simulink model "ChuaMultipleSynch_MPC_2"  (R2014b)
settings: Solver=ode4  StartTime=0.0  StopTime=T  FixedStep=Ts  RelTol=1e-8
values from neighbouring files (symbols this model uses):
  mpc = MPCController(model, N)    [main_mpc.m]
  x0 = [0.02;0.05;0.04;0.0;1.0;0.0]    [PlotEig.m]    (also in main_mpc.m; main_sim.m)
undefined symbols (not defined in the file or in its folder): MPC_Controller
settings Model: Creator=gianni  LastModifiedBy=Gianni

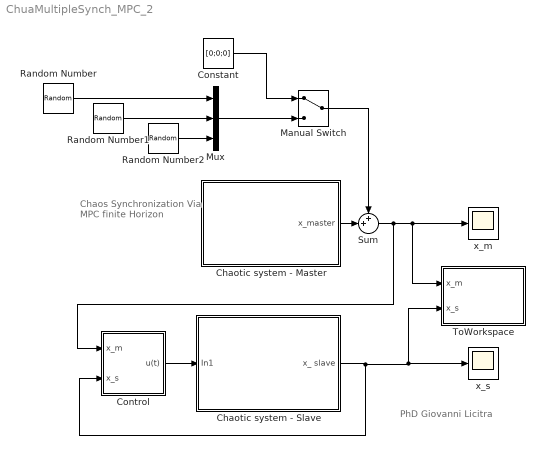
== system ChuaMultipleSynch_MPC_2 ==
  note: PhD Giovanni Licitra
  note: Chaos Synchronization
      | Via MPC finite Horizon
  Chaotic system - Master : Subsystem
      mask Display: image('Chaos.jpg')
  Chaotic system - Slave : Subsystem
      mask Display: image('Chaos.jpg')
  Constant : Constant  Value=[0;0;0]
  Control : Subsystem
  Manual Switch : ManualSwitch
  Mux : Mux  Inputs=3
  Random Number : RandomNumber  Variance=0.002
  Random Number1 : RandomNumber  Variance=0.002
  Random Number2 : RandomNumber  Variance=0.002
  Sum : Sum  Inputs=++|
  ToWorkspace : Subsystem
  x_m : Scope
      settings: YMin=-0.4  YMax=0.4
  x_s : Scope
      settings: YMin=-2
  wires:
  Control/1(u(t)) -> Chaotic system - Slave/1(In1)
  Sum/1 -> ToWorkspace/1(x_m), x_m/1, Control/1(x_m)
  Chaotic system - Slave/1(x_ slave) -> Control/2(x_s), ToWorkspace/2(x_s), x_s/1
  Mux/1 -> Manual Switch/2
  Chaotic system - Master/1(x_master) -> Sum/2
  Manual Switch/1 -> Sum/1
  Random Number/1 -> Mux/1
  Random Number1/1 -> Mux/2
  Random Number2/1 -> Mux/3
  Constant/1 -> Manual Switch/1

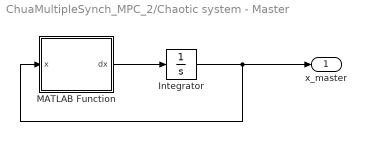
== system ChuaMultipleSynch_MPC_2/Chaotic system - Master ==
  Integrator : Integrator  InitialCondition=x0([1:3])
  MATLAB Function : MATLAB Function  TreatAsAtomicUnit=on
  x_master : Outport
  wires:
  Integrator/1 -> x_master/1, MATLAB Function/1(x)
  MATLAB Function/1(dx) -> Integrator/1

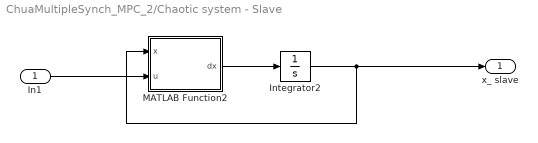
== system ChuaMultipleSynch_MPC_2/Chaotic system - Slave ==
  In1 : Inport
  Integrator2 : Integrator  InitialCondition=x0([4:6])
  MATLAB Function2 : MATLAB Function  TreatAsAtomicUnit=on
  x_ slave : Outport
  wires:
  MATLAB Function2/1(dx) -> Integrator2/1
  In1/1 -> MATLAB Function2/2(u)
  Integrator2/1 -> x_ slave/1, MATLAB Function2/1(x)

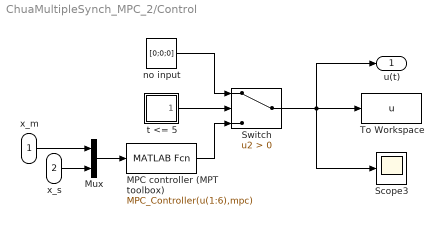
== system ChuaMultipleSynch_MPC_2/Control ==
  x_m : Inport
  x_s : Inport  Port=2
  MPC controller (MPT toolbox) : MATLABFcn  MATLABFcn=MPC_Controller(u(1:6),mpc)
  Mux : Mux  Inputs=2
  Scope3 : Scope
      settings: YMin=-20  YMax=20  SaveName=ScopeData3
  Switch : Switch  Criteria=u2 > Threshold
  To Workspace : ToWorkspace  VariableName=u  SaveFormat=Timeseries  SampleTime=-1
  no input : Constant  Value=[0;0;0]
  t <= 5 : Subsystem
  u(t) : Outport
  wires:
  x_s/1 -> Mux/2
  x_m/1 -> Mux/1
  t <= 5/1(t <= 3) -> Switch/2
  no input/1 -> Switch/1
  Switch/1 -> Scope3/1, To Workspace/1, u(t)/1
  MPC controller (MPT toolbox)/1 -> Switch/3
  Mux/1 -> MPC controller (MPT toolbox)/1

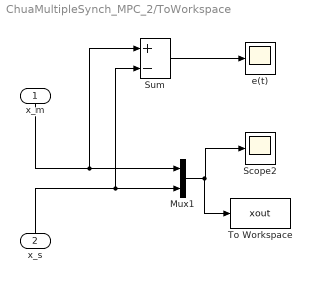
== system ChuaMultipleSynch_MPC_2/ToWorkspace ==
  x_m : Inport
  x_s : Inport  Port=2
  Mux1 : Mux  Inputs=2
  Scope2 : Scope
      settings: YMin=-3  SaveName=ScopeData2
  Sum : Sum  Inputs=+-
  To Workspace : ToWorkspace  VariableName=xout  SaveFormat=Timeseries  SampleTime=-1
  e(t) : Scope
      settings: YMin=-6  YMax=3  SaveName=ScopeData4
  wires:
  Mux1/1 -> To Workspace/1, Scope2/1
  x_s/1 -> Sum/2, Mux1/2
  x_m/1 -> Sum/1, Mux1/1
  Sum/1 -> e(t)/1

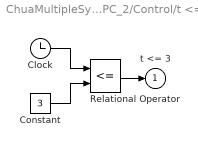
== system ChuaMultipleSynch_MPC_2/Control/t <= 5 ==
  Clock : Clock
  Constant : Constant  Value=3
  Relational Operator : RelationalOperator  Operator=<=  InputSameDT=on
  t <= 3 : Outport  InitialOutput=0
  wires:
  Constant/1 -> Relational Operator/2
  Clock/1 -> Relational Operator/1
  Relational Operator/1 -> t <= 3/1

== matlab function ChuaMultipleSynch_MPC_2/Chaotic system - Master/MATLAB Function ==
  data: x input; dx output
function dx = ode(x)                             
    alpha = 15.6;beta = 28;m0 = -1.143;m1 = -0.714; % master system parameter 
    x1 = x(1);y1 = x(2);z1 = x(3);     % master sys states    
    f_x1 = m1*x1+0.5*(m0-m1)*(abs(x1+1)-abs(x1-1)); % non linearita master
    dx = [alpha*(y1-x1-f_x1);% 
          x1 - y1+ z1;
          -beta*y1];    
end

== matlab function ChuaMultipleSynch_MPC_2/Chaotic system - Slave/MATLAB Function2 ==
  data: x input; dx output; u input
function dx = ode(x,u)                             
    a = 28;b = 10;c = 8/3;             % slave system parameter    
    x2 = x(1);y2 = x(2);z2 = x(3);     % slave sys states
    ux = u(1);uy = u(2); uz = u(3);    % control to slave system
        
    dx = [b*(y2-x2)+ux;
          x2*(a-z2)-y2+uy;
          x2*y2-c*z2+uz];
end
